simulink model "AtuadorHidraulicoLinear"  (R2015a)
settings: Solver=ode45  StartTime=0.0  StopTime=10.0  RelTol=1e-3
libraries: simulink x4
settings Model: Creator=Wagner  LastModifiedBy=Wagner

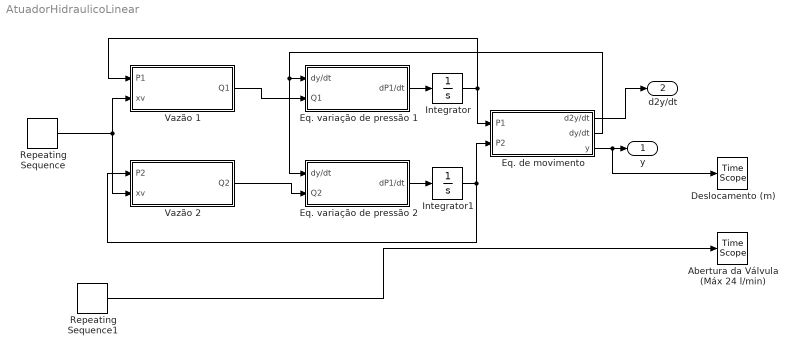
== system AtuadorHidraulicoLinear ==
  Abertura da Válvula (Máx 24 l/min) : TimeScope
  Deslocamento (m) : TimeScope
  Eq. de movimento : Subsystem
  Eq. variação de pressão 1 : Subsystem
  Eq. variação de pressão 2 : Subsystem
  Integrator : Integrator
  Integrator1 : Integrator
  Repeating Sequence : simulink/Sources/Repeating Sequence  rep_seq_t=[0 1 1.0001 2]  rep_seq_y=[4.8 4.8 0 0]
  Repeating Sequence1 : simulink/Sources/Repeating Sequence  rep_seq_t=[0 1 1.0001 2]  rep_seq_y=[4.8 4.8 0 0]
  Vazão 1 : Subsystem
  Vazão 2 : Subsystem
  y : Outport
  d2y/dt : Outport  Port=2
  wires:
  Repeating Sequence/1 -> Vazão 2/2(xv), Vazão 1/2(xv)
  Vazão 2/1(Q2) -> Eq. variação de pressão 2/2(Q2)
  Eq. variação de pressão 1/1(dP1/dt) -> Integrator/1
  Eq. variação de pressão 2/1(dP1/dt) -> Integrator1/1
  Integrator1/1 -> Vazão 2/1(P2), Eq. de movimento/2(P2)
  Integrator/1 -> Eq. de movimento/1(P1), Vazão 1/1(P1)
  Eq. de movimento/2(dy/dt) -> Eq. variação de pressão 1/1(dy/dt), Eq. variação de pressão 2/1(dy/dt)
  Eq. de movimento/3(y) -> Deslocamento (m)/1, y/1
  Eq. de movimento/1(d2y/dt) -> d2y/dt/1
  Vazão 1/1(Q1) -> Eq. variação de pressão 1/2(Q1)
  Repeating Sequence1/1 -> Abertura da Válvula (Máx 24 l/min)/1

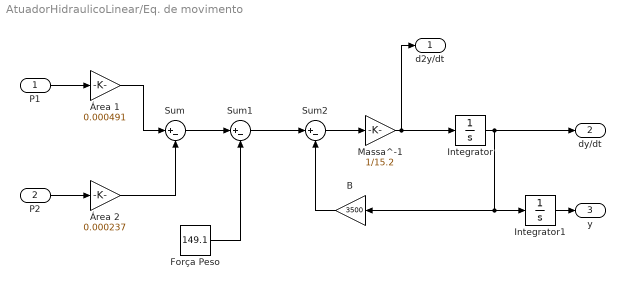
== system AtuadorHidraulicoLinear/Eq. de movimento ==
  P1 : Inport
  P2 : Inport  Port=2
  B : Gain  Gain=3500
  Força Peso : Constant  Value=149.1
  Integrator : Integrator
  Integrator1 : Integrator
  Massa^-1 : Gain  Gain=1/15.2
  Sum : Sum  Inputs=|+-
  Sum1 : Sum  Inputs=|+-
  Sum2 : Sum  Inputs=|+-
  Área 1 : Gain  Gain=0.000491
  Área 2 : Gain  Gain=0.000237
  d2y/dt : Outport
  dy/dt : Outport  Port=2
  y : Outport  Port=3
  wires:
  P1/1 -> Área 1/1
  Área 1/1 -> Sum/1
  P2/1 -> Área 2/1
  Área 2/1 -> Sum/2
  Sum/1 -> Sum1/1
  Sum1/1 -> Sum2/1
  Sum2/1 -> Massa^-1/1
  Massa^-1/1 -> d2y/dt/1, Integrator/1
  B/1 -> Sum2/2
  Integrator/1 -> B/1, Integrator1/1, dy/dt/1
  Integrator1/1 -> y/1
  Força Peso/1 -> Sum1/2

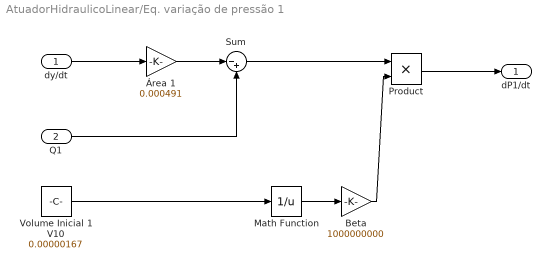
== system AtuadorHidraulicoLinear/Eq. variação de pressão 1 ==
  dy/dt : Inport
  Q1 : Inport  Port=2
  Beta : Gain  Gain=1000000000
  Math Function : Math  Operator=reciprocal  RndMeth=Zero  SaturateOnIntegerOverflow=on
  Product : Product
  Sum : Sum  Inputs=|-+
  Volume Inicial 1 V10 : Constant  Value=0.00000167
  Área 1 : Gain  Gain=0.000491
  dP1/dt : Outport
  wires:
  dy/dt/1 -> Área 1/1
  Área 1/1 -> Sum/1
  Q1/1 -> Sum/2
  Sum/1 -> Product/1
  Beta/1 -> Product/2
  Math Function/1 -> Beta/1
  Product/1 -> dP1/dt/1
  Volume Inicial 1 V10/1 -> Math Function/1

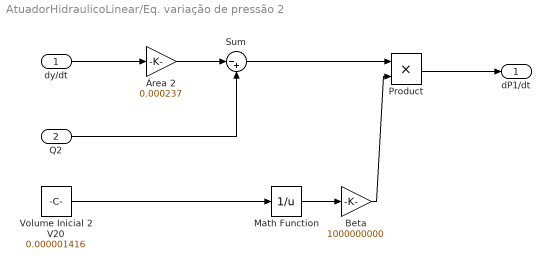
== system AtuadorHidraulicoLinear/Eq. variação de pressão 2 ==
  dy/dt : Inport
  Q2 : Inport  Port=2
  Beta : Gain  Gain=1000000000
  Math Function : Math  Operator=reciprocal  RndMeth=Zero  SaturateOnIntegerOverflow=on
  Product : Product
  Sum : Sum  Inputs=|-+
  Volume Inicial 2 V20 : Constant  Value=0.000001416
  Área 2 : Gain  Gain=0.000237
  dP1/dt : Outport
  wires:
  dy/dt/1 -> Área 2/1
  Área 2/1 -> Sum/1
  Q2/1 -> Sum/2
  Sum/1 -> Product/1
  Beta/1 -> Product/2
  Math Function/1 -> Beta/1
  Product/1 -> dP1/dt/1
  Volume Inicial 2 V20/1 -> Math Function/1

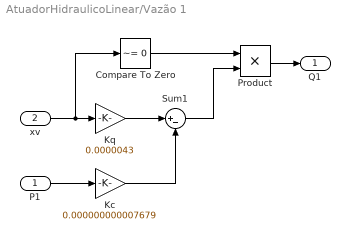
== system AtuadorHidraulicoLinear/Vazão 1 ==
  P1 : Inport
  xv : Inport  Port=2
  Compare To Zero : simulink/Logic and Bit Operations/Compare To Zero  relop=~=  OutDataTypeStr=boolean
  Kc : Gain  Gain=0.000000000007679
  Kq : Gain  Gain=0.0000043
  Product : Product
  Sum1 : Sum  Inputs=|+-
  Q1 : Outport
  wires:
  Kq/1 -> Sum1/1
  xv/1 -> Compare To Zero/1, Kq/1
  P1/1 -> Kc/1
  Kc/1 -> Sum1/2
  Product/1 -> Q1/1
  Sum1/1 -> Product/2
  Compare To Zero/1 -> Product/1

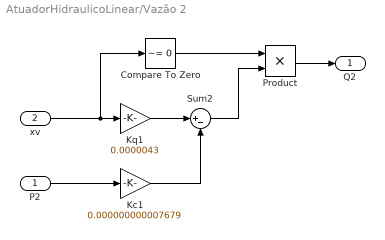
== system AtuadorHidraulicoLinear/Vazão 2 ==
  P2 : Inport
  xv : Inport  Port=2
  Compare To Zero : simulink/Logic and Bit Operations/Compare To Zero  relop=~=  OutDataTypeStr=boolean
  Kc1 : Gain  Gain=0.000000000007679
  Kq1 : Gain  Gain=0.0000043
  Product : Product
  Sum2 : Sum  Inputs=|+-
  Q2 : Outport
  wires:
  Kq1/1 -> Sum2/1
  xv/1 -> Compare To Zero/1, Kq1/1
  P2/1 -> Kc1/1
  Kc1/1 -> Sum2/2
  Product/1 -> Q2/1
  Sum2/1 -> Product/2
  Compare To Zero/1 -> Product/1
